simulink model "smartDirectServoCartesian"  (R2018a)
settings: Solver=FixedStepAuto  StartTime=0.0  StopTime=100.0  RelTol=1e-3
libraries: dspsrcs4 x2, dspnetwork x1, sldrtlib x1
settings Model: Creator=ronnie  LastModifiedBy=user

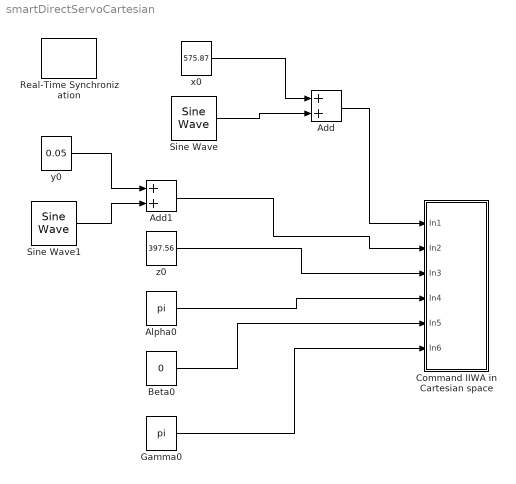
== system smartDirectServoCartesian ==
  Add : Sum
  Add1 : Sum
  Alpha0 : Constant  Value=pi  VectorParams1D=off  SampleTime=1/1000
  Beta0 : Constant  Value=0  VectorParams1D=off  SampleTime=1/1000
  Command IIWA in Cartesian space : Subsystem
  Gamma0 : Constant  Value=pi  VectorParams1D=off  SampleTime=1/1000
  Real-Time Synchronization : sldrtlib/Real-Time Synchronization  SampleTime=0.01  MaxMissedTicks=10  ShowMissedTicks=off  YieldWhenWaiting=off
  Sine Wave : dspsrcs4/Sine Wave  Amplitude=80  Frequency=0.15  Phase=0  SampleMode=Discrete  OutComplex=Real  CompMethod=Trigonometric fcn  TableSize=Speed  SampleTime=1/1000  SamplesPerFrame=1  ResetState=Restart at time zero  OutputFrames=off  dataType=double  wordLen=16  udDataType=sfix(16)  fracBitsMode=Best precision  numFracBits=15  OutDataTypeStr=double  LastOutDataTypeStr=double
  Sine Wave1 : dspsrcs4/Sine Wave  Amplitude=75  Frequency=0.2  Phase=0  SampleMode=Discrete  OutComplex=Real  CompMethod=Trigonometric fcn  TableSize=Speed  SampleTime=1/1000  SamplesPerFrame=1  ResetState=Restart at time zero  OutputFrames=off  dataType=double  wordLen=16  udDataType=sfix(16)  fracBitsMode=Best precision  numFracBits=15  OutDataTypeStr=double  LastOutDataTypeStr=double
  x0 : Constant  Value=575.87  VectorParams1D=off  SampleTime=1/1000
  y0 : Constant  Value=0.05  VectorParams1D=off  SampleTime=1/1000
  z0 : Constant  Value=397.56  VectorParams1D=off  SampleTime=1/1000
  wires:
  Beta0/1 -> Command IIWA in Cartesian space/5(In5)
  Alpha0/1 -> Command IIWA in Cartesian space/4(In4)
  z0/1 -> Command IIWA in Cartesian space/3(In3)
  Sine Wave/1 -> Add/2
  x0/1 -> Add/1
  Add/1 -> Command IIWA in Cartesian space/1(In1)
  Add1/1 -> Command IIWA in Cartesian space/2(In2)
  y0/1 -> Add1/1
  Sine Wave1/1 -> Add1/2
  Gamma0/1 -> Command IIWA in Cartesian space/6(In6)

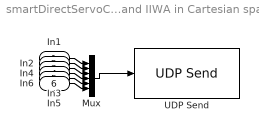
== system smartDirectServoCartesian/Command IIWA in Cartesian space ==
  In1 : Inport
  In2 : Inport  Port=2
  In3 : Inport  Port=3
  In4 : Inport  Port=4
  In5 : Inport  Port=5
  In6 : Inport  Port=6
  Mux : Mux  Inputs=6
  UDP Send : dspnetwork/UDP Send  remoteURL='172.31.1.147'  remotePort=30002  localURL='0.0.0.0'  localPortSource=Automatically determine  localPort=-1  sampletime=-1  blockPlatform=[]  separateLengthPort=0
      settings: SourceProductName=DSP System Toolbox  SourceProductBaseCode=DS
  wires:
  Mux/1 -> UDP Send/1
  In3/1 -> Mux/3
  In5/1 -> Mux/5
  In2/1 -> Mux/2
  In1/1 -> Mux/1
  In6/1 -> Mux/6
  In4/1 -> Mux/4
